simulink model "Openloop_3DOF_Simulator"  (R2018a)
settings: Solver=ode4  StartTime=0.0  StopTime=10  FixedStep=1e-2  RelTol=1e-3  EnableMultiTasking=on
settings Model: Creator=yashwanth  LastModifiedBy=ynakka
settings DataIOCC: LimitDataPoints=on
settings OptimizationCC: LifeSpan=inf
settings DebuggingCC: AllowSymbolicDim=off  SFUnexpectedBacktrackingDiag=warning  SFNoUnconditionalDefaultTransitionDiag=warning  SFExecutionAtInitializationDiag=none
settings ModelReferenceCC: PropagateSignalLabelsOutOfModel=off
settings CodeAppCC: StateflowObjectComments=on
settings GRTTargetCC: TargetLangStandard=C89/C90 (ANSI)
settings ConfigComp: CovMetricSettings=dw  CovHtmlReporting=on  CovSaveCumulativeToWorkspaceVar=on  CovSaveSingleToWorkspaceVar=on  CovExternalEMLEnable=off

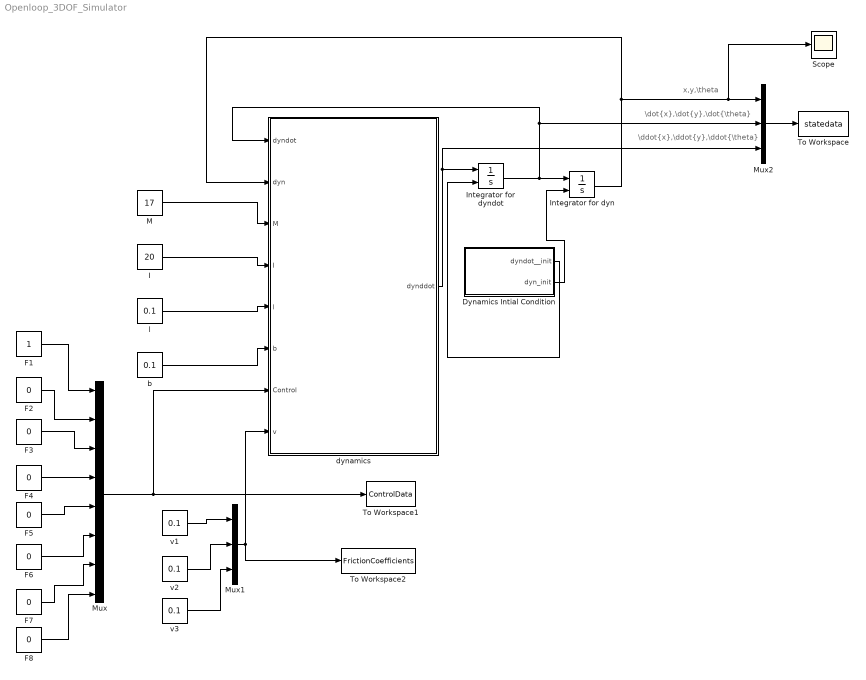
== system Openloop_3DOF_Simulator ==
  note: x,y,\theta
  note: \dot{x},\dot{y},\dot{\theta}
  note: \ddot{x},\ddot{y},\ddot{\theta}
  Dynamics Intial Condition : Subsystem
  F1 : Constant  VectorParams1D=off
  F{2..8} (7 alike) : Constant  Value=0  VectorParams1D=off
  I : Constant  Value=20  VectorParams1D=off
  Integrator for dyn : Integrator  InitialConditionSource=external  InitialCondition=-0.1  AbsoluteTolerance=1e-3
  Integrator for dyndot : Integrator  InitialConditionSource=external  InitialCondition=-0.1  UpperSaturationLimit=1e20  LowerSaturationLimit=-1e20  AbsoluteTolerance=1e-10
  M : Constant  Value=17  VectorParams1D=off
  Mux : Mux  Inputs=8
  Mux1 : Mux  Inputs=3
  Mux2 : Mux  Inputs=3
  Scope : Scope
  To Workspace : ToWorkspace  VariableName=statedata  SaveFormat=Timeseries  SampleTime=-1
  To Workspace1 : ToWorkspace  VariableName=ControlData  SaveFormat=Timeseries  SampleTime=-1
  To Workspace2 : ToWorkspace  VariableName=FrictionCoefficients  SaveFormat=Timeseries  SampleTime=-1
  b : Constant  Value=0.1  VectorParams1D=off
  dynamics : MATLAB Function  TreatAsAtomicUnit=on
  l : Constant  Value=0.1  VectorParams1D=off
  v1 : Constant  Value=0.1  VectorParams1D=off
  v2 : Constant  Value=0.1  VectorParams1D=off
  v3 : Constant  Value=0.1  VectorParams1D=off
  wires:
  M/1 -> dynamics/3(M)
  Integrator for dyndot/1 -> Mux2/2, dynamics/1(dyndot), Integrator for dyn/1
  Integrator for dyn/1 -> Scope/1, Mux2/1, dynamics/2(dyn)
  dynamics/1(dynddot) -> Integrator for dyndot/1, Mux2/3
  Dynamics Intial Condition/1(dyndot__init) -> Integrator for dyndot/2
  Dynamics Intial Condition/2(dyn_init) -> Integrator for dyn/2
  I/1 -> dynamics/4(I)
  l/1 -> dynamics/5(l)
  b/1 -> dynamics/6(b)
  Mux/1 -> dynamics/7(Control), To Workspace1/1
  F7/1 -> Mux/7
  F6/1 -> Mux/6
  F5/1 -> Mux/5
  F4/1 -> Mux/4
  F3/1 -> Mux/3
  F2/1 -> Mux/2
  F1/1 -> Mux/1
  F8/1 -> Mux/8
  v1/1 -> Mux1/1
  v2/1 -> Mux1/2
  v3/1 -> Mux1/3
  Mux1/1 -> dynamics/8(v), To Workspace2/1
  Mux2/1 -> To Workspace/1

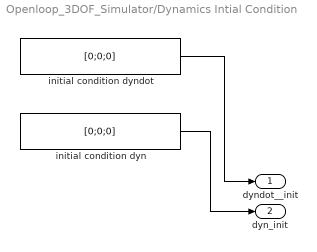
== system Openloop_3DOF_Simulator/Dynamics Intial Condition ==
  initial condition dyn : Constant  Value=[0;0;0]
  initial condition dyndot : Constant  Value=[0;0;0]
  dyndot__init : Outport
  dyn_init : Outport  Port=2
  wires:
  initial condition dyn/1 -> dyn_init/1
  initial condition dyndot/1 -> dyndot__init/1

== matlab function Openloop_3DOF_Simulator/dynamics ==
  data: dyndot input; dyn input; dynddot output; M input; I input; l input; b input; Control input; v input
function dynddot  = fcn(dyndot,dyn,M,I,l,b,Control,v)

% x = dyn(1);
% y = dyn(2);
% theta = dyn(3);

c = cos(dyn(3))/M;
s = sin(dyn(3))/M;
ll = l/(2*I);
bb = b/(2*I);
R1 = [-c -c s s c c -s -s];
R2 = [-s -s -c -c s s c c];
R3 = [-ll ll -bb bb -ll ll -bb bb];

Matrix = [R1;R2;R3];

dynddot= Matrix*Control - [v(1)/M 0 0;0 v(2)/M 0;0 0 v(3)/(2*I)]*dyndot;
